simulink model "topProject"  (R2016b)
settings: Solver=ode45  StartTime=0.0  StopTime=40.0  RelTol=1e-3  EnableMultiTasking=on
libraries: simulink x3, powerlib x1
settings Model: Creator=Aluno IC  LastModifiedBy=icaro
settings DataIOCC: LimitDataPoints=on  SaveFormat=Array
settings OptimizationCC: LifeSpan=inf
settings DebuggingCC: SFUnexpectedBacktrackingDiag=warning  SFNoUnconditionalDefaultTransitionDiag=warning  SFExecutionAtInitializationDiag=none
settings HardwareCC: ProdBitPerPointer=32  ProdBitPerSizeT=32  ProdBitPerPtrDiffT=32  ProdLargestAtomicFloat=None  ProdIntDivRoundTo=Undefined  ProdEndianess=Unspecified  ProdWordSize=32  ProdHWDeviceType=32-bit Generic
settings ModelReferenceCC: PropagateSignalLabelsOutOfModel=off
settings GRTTargetCC: TargetLangStandard=C89/C90 (ANSI)  GeneratePreprocessorConditionals=Disable all
settings ConfigComp: CovMetricSettings=dw  CovHtmlReporting=on  CovSaveCumulativeToWorkspaceVar=on  CovSaveSingleToWorkspaceVar=on  CovExternalEMLEnable=off

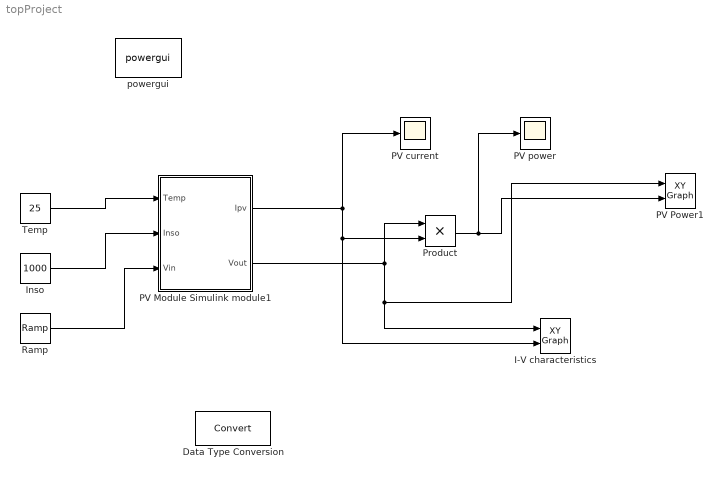
== system topProject ==
  Data Type Conversion : DataTypeConversion
  I-V characteristics : simulink/Sinks/XY Graph  xmin=-1  xmax=40  ymin=-1  ymax=40  st=-1
  Inso : Constant  Value=1000
  PV Module Simulink module1 : Subsystem
  PV Power1 : simulink/Sinks/XY Graph  xmin=-1  xmax=40  ymin=-1  ymax=40  st=-1
  PV current : Scope
  "PV power " : Scope
  Product : Product
  Ramp : simulink/Sources/Ramp  slope=1  start=0  X0=0
  Temp : Constant  Value=25
  powergui : powerlib/powergui  Priority=1  SimulationMode=Continuous  SolverType=Tustin/Backward Euler (TBE)  SampleTime=50e-6  frequency=60  SPID=off  DisableSnubberDevices=off  DisableRonSwitches=off  DisableVfSwitches=off  SwTol=0  DisplayEquations=off  Interpol=off  ExternalGateDelay=off  methode=off  Ts=10  FunctionMessages=off  echomessages=off  HookPort=off  EnableUseOfTLC=off  x0status=blocks  frequencyindice=0  Pbase=100e6  ErrMax=1e-4  Iterations=50  UnitsV=kV  UnitsW=MW  buscounter=0  RestoreLinks=warning  ResistiveCurrentMeasurement=off  Frange=[0:2:500]  Ylog=off  Xlog=on  ShowGrid=off  save=off  variable=ZData  structure=0  ZoomFFT=off  StartTime=0.0  cycles=1  DisplayStyle=1  fundamental=60  FreqAxis=off  MaxFrequency=1000  frequencyindicesteady=1  RmsSteady=1  display=off
  wires:
  Ramp/1 -> PV Module Simulink module1/3(Vin)
  Inso/1 -> PV Module Simulink module1/2(Inso)
  Temp/1 -> PV Module Simulink module1/1(Temp)
  PV Module Simulink module1/1(Ipv) -> I-V characteristics/2, Product/2, PV current/1
  Product/1 -> "PV power "/1, PV Power1/2
  PV Module Simulink module1/2(Vout) -> I-V characteristics/1, PV Power1/1, Product/1

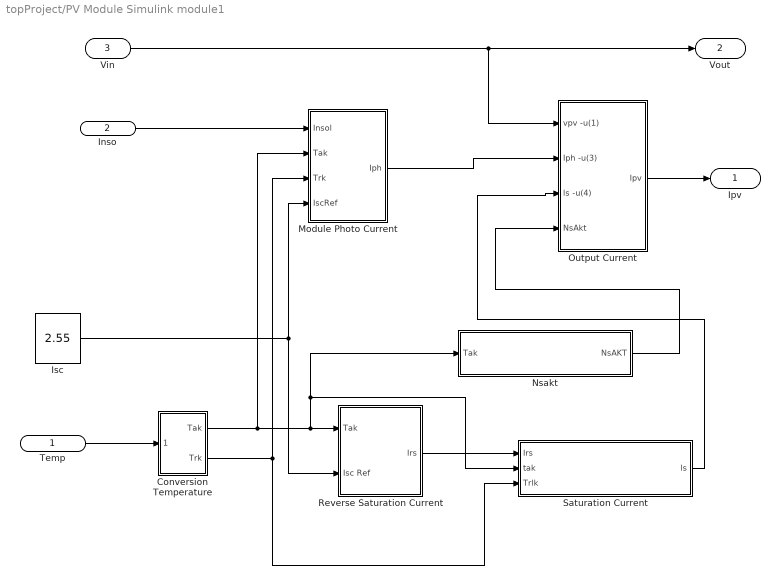
== system topProject/PV Module Simulink module1 ==
  Temp : Inport
  Inso : Inport  Port=2
  Vin : Inport  Port=3
  Conversion Temperature : Subsystem
  Isc : Constant  Value=2.55
  Module Photo Current : Subsystem
  "Nsakt " : Subsystem
  "Output Current " : Subsystem
  Reverse Saturation Current : Subsystem
  Saturation Current : Subsystem
  Ipv : Outport
  Vout : Outport  Port=2
  wires:
  Conversion Temperature/1("Tak ") -> Module Photo Current/2("Tak "), "Nsakt "/1(Tak), Saturation Current/2(tak), Reverse Saturation Current/1(Tak)
  Saturation Current/1(ls) -> "Output Current "/3(ls -u(4))
  "Nsakt "/1("NsAKT ") -> "Output Current "/4(NsAkt)
  Module Photo Current/1(Iph) -> "Output Current "/2(Iph -u(3))
  Conversion Temperature/2(Trk) -> Saturation Current/3(Trlk), Module Photo Current/3("Trk ")
  Temp/1 -> Conversion Temperature/1("Top ")
  Inso/1 -> Module Photo Current/1(Insol)
  Reverse Saturation Current/1(Irs) -> Saturation Current/1("Irs ")
  Vin/1 -> Vout/1, "Output Current "/1(vpv -u(1))
  Isc/1 -> Module Photo Current/4(IscRef), Reverse Saturation Current/2(Isc Ref)
  "Output Current "/1(Ipv) -> Ipv/1

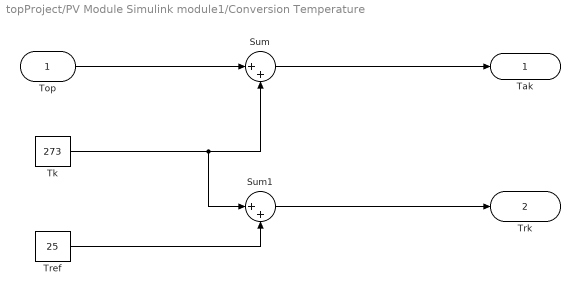
== system topProject/PV Module Simulink module1/Conversion Temperature ==
  "Top " : Inport
  Sum : Sum  Inputs=|++
  Sum1 : Sum  Inputs=|++
  Tk : Constant  Value=273
  Tref : Constant  Value=25
  "Tak " : Outport
  Trk : Outport  Port=2
  wires:
  Sum1/1 -> Trk/1
  Tref/1 -> Sum1/2
  "Top "/1 -> Sum/1
  Tk/1 -> Sum1/1, Sum/2
  Sum/1 -> "Tak "/1

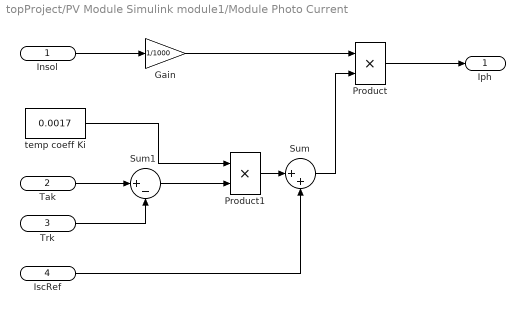
== system topProject/PV Module Simulink module1/Module Photo Current ==
  Insol : Inport
  "Tak " : Inport  Port=2
  "Trk " : Inport  Port=3
  IscRef : Inport  Port=4
  Gain : Gain  Gain=1/1000
  Product : Product
  Product1 : Product
  Sum : Sum  Inputs=|++
  Sum1 : Sum  Inputs=|+-
  temp coeff Ki : Constant  Value=0.0017
  Iph : Outport
  wires:
  IscRef/1 -> Sum/2
  Gain/1 -> Product/1
  Sum1/1 -> Product1/2
  Product1/1 -> Sum/1
  Product/1 -> Iph/1
  "Tak "/1 -> Sum1/1
  Sum/1 -> Product/2
  "Trk "/1 -> Sum1/2
  temp coeff Ki/1 -> Product1/1
  Insol/1 -> Gain/1

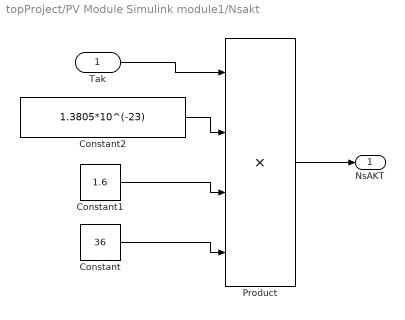
== system topProject/PV Module Simulink module1/Nsakt  ==
  Tak : Inport
  Constant : Constant  Value=36
  Constant1 : Constant  Value=1.6
  Constant2 : Constant  Value=1.3805*10^(-23)
  Product : Product  Inputs=4
  "NsAKT " : Outport
  wires:
  Product/1 -> "NsAKT "/1
  Constant2/1 -> Product/2
  Constant1/1 -> Product/3
  Constant/1 -> Product/4
  Tak/1 -> Product/1

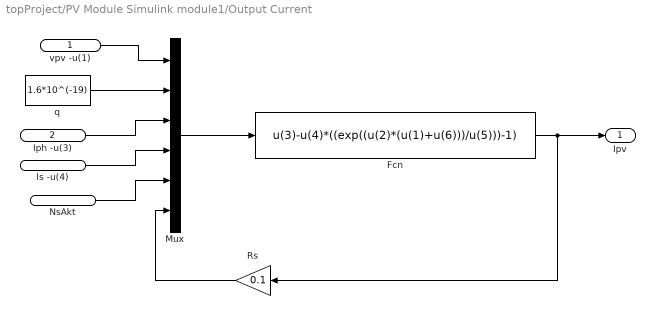
== system topProject/PV Module Simulink module1/Output Current  ==
  vpv -u(1) : Inport
  Iph -u(3) : Inport  Port=2
  ls -u(4) : Inport  Port=3
  NsAkt : Inport  Port=4
  Fcn : Fcn  Expr=u(3)-u(4)*((exp((u(2)*(u(1)+u(6)))/u(5)))-1)
  Mux : Mux  Inputs=6
  Rs : Gain  Gain=0.1
  q : Constant  Value=1.6*10^(-19)
  Ipv : Outport
  wires:
  q/1 -> Mux/2
  Rs/1 -> Mux/6
  Iph -u(3)/1 -> Mux/3
  ls -u(4)/1 -> Mux/4
  NsAkt/1 -> Mux/5
  vpv -u(1)/1 -> Mux/1
  Fcn/1 -> Ipv/1, Rs/1
  Mux/1 -> Fcn/1

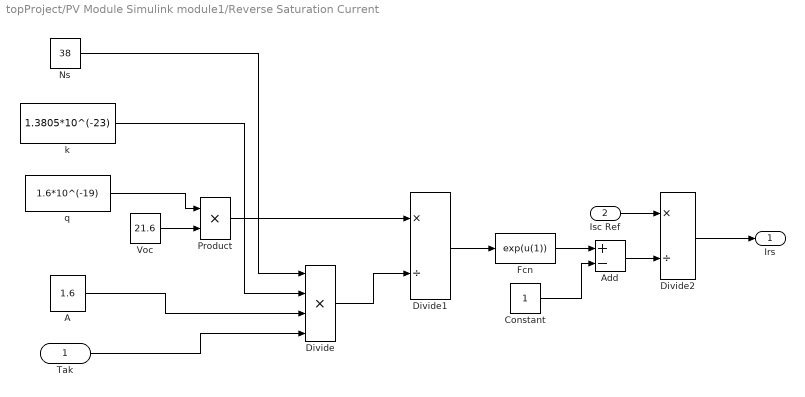
== system topProject/PV Module Simulink module1/Reverse Saturation Current ==
  Tak : Inport
  Isc Ref : Inport  Port=2
  A : Constant  Value=1.6
  Add : Sum  Inputs=+-
  Constant : Constant
  Divide : Product  Inputs=4
  Divide1 : Product  Inputs=*/
  Divide2 : Product  Inputs=*/
  Fcn : Fcn  Expr=exp(u(1))
  Ns : Constant  Value=38
  Product : Product
  Voc : Constant  Value=21.6
  k : Constant  Value=1.3805*10^(-23)
  q : Constant  Value=1.6*10^(-19)
  Irs : Outport
  wires:
  Divide2/1 -> Irs/1
  Ns/1 -> Divide/1
  Isc Ref/1 -> Divide2/1
  Divide1/1 -> Fcn/1
  Product/1 -> Divide1/1
  k/1 -> Divide/2
  A/1 -> Divide/3
  Divide/1 -> Divide1/2
  Tak/1 -> Divide/4
  Add/1 -> Divide2/2
  Fcn/1 -> Add/1
  Constant/1 -> Add/2
  q/1 -> Product/1
  Voc/1 -> Product/2

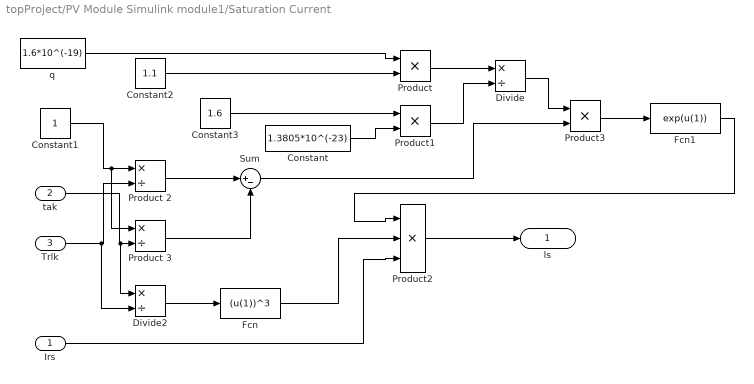
== system topProject/PV Module Simulink module1/Saturation Current ==
  "Irs " : Inport
  tak : Inport  Port=2
  Trlk : Inport  Port=3
  Constant : Constant  Value=1.3805*10^(-23)
  Constant1 : Constant
  Constant2 : Constant  Value=1.1
  Constant3 : Constant  Value=1.6
  Divide : Product  Inputs=*/
  Divide2 : Product  Inputs=*/
  Fcn : Fcn  Expr=(u(1))^3
  Fcn1 : Fcn  Expr=exp(u(1))
  Product : Product
  Product 2 : Product  Inputs=*/
  Product 3 : Product  Inputs=*/
  Product1 : Product
  Product2 : Product  Inputs=3
  Product3 : Product
  Sum : Sum  Inputs=|+-
  q : Constant  Value=1.6*10^(-19)
  ls : Outport
  wires:
  Constant2/1 -> Product/2
  Product3/1 -> Fcn1/1
  "Irs "/1 -> Product2/3
  q/1 -> Product/1
  Fcn/1 -> Product2/2
  Divide2/1 -> Fcn/1
  Product 2/1 -> Sum/1
  Product 3/1 -> Sum/2
  Product2/1 -> ls/1
  Product/1 -> Divide/1
  Constant3/1 -> Product1/1
  Sum/1 -> Product3/2
  Product1/1 -> Divide/2
  Constant/1 -> Product1/2
  Fcn1/1 -> Product2/1
  Divide/1 -> Product3/1
  Trlk/1 -> Product 2/2, Divide2/2
  tak/1 -> Divide2/1, Product 3/2
  Constant1/1 -> Product 3/1, Product 2/1
